simulink model "DSM_2"  (R2024b)
settings: Solver=VariableStepAuto  StartTime=0.0  StopTime=8e-3  RelTol=1e-3
undefined symbols (not defined in the file or in its folder): dspblkCoreblockFVToolHelper, gcbh
libraries: simulink x1
settings Model: Creator=peggy  LastModifiedBy=peggy

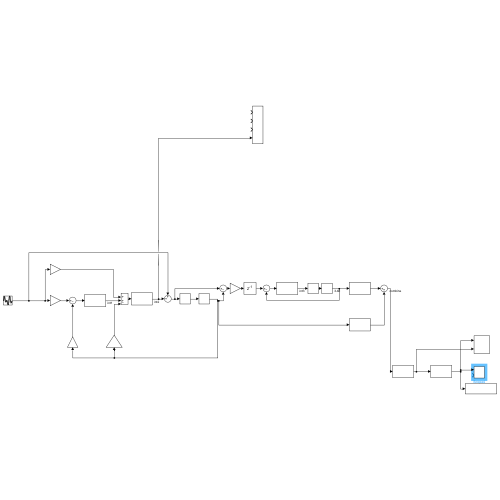
[thumbnail: Simulink's stored preview of the top-level diagram]
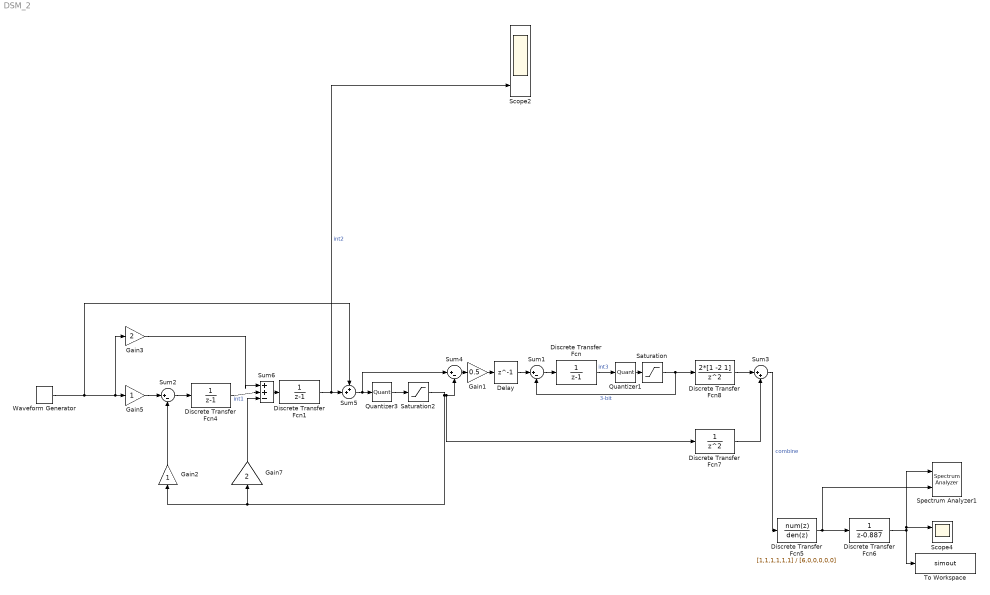
== system DSM_2 ==
  Delay : Delay  DelayLength=1  InitialCondition=0
  Discrete Transfer Fcn : DiscreteTransferFcn  LoadFcn=dspblkCoreblockFVToolHelper(gcbh,'load');  Denominator=[1 -1]
      settings: CopyFcn=dspblkCoreblockFVToolHelper(gcbh,'copy');  DeleteFcn=dspblkCoreblockFVToolHelper(gcbh,'close');  ModelCloseFcn=dspblkCoreblockFVToolHelper(gcbh,'close');  PreSaveFcn=dspblkCoreblockFVToolHelper(gcbh,'presave');  PostSaveFcn=dspblkCoreblockFVToolHelper(gcbh,'postsave');  CloseFcn=dspblkCoreblockFVToolHelper(gcbh,'close');
  Discrete Transfer Fcn1 : DiscreteTransferFcn  LoadFcn=dspblkCoreblockFVToolHelper(gcbh,'load');  Denominator=[1 -1]
      settings: CopyFcn=dspblkCoreblockFVToolHelper(gcbh,'copy');  DeleteFcn=dspblkCoreblockFVToolHelper(gcbh,'close');  ModelCloseFcn=dspblkCoreblockFVToolHelper(gcbh,'close');  PreSaveFcn=dspblkCoreblockFVToolHelper(gcbh,'presave');  PostSaveFcn=dspblkCoreblockFVToolHelper(gcbh,'postsave');  CloseFcn=dspblkCoreblockFVToolHelper(gcbh,'close');
  Discrete Transfer Fcn4 : DiscreteTransferFcn  LoadFcn=dspblkCoreblockFVToolHelper(gcbh,'load');  Denominator=[1 -1]
      settings: CopyFcn=dspblkCoreblockFVToolHelper(gcbh,'copy');  DeleteFcn=dspblkCoreblockFVToolHelper(gcbh,'close');  ModelCloseFcn=dspblkCoreblockFVToolHelper(gcbh,'close');  PreSaveFcn=dspblkCoreblockFVToolHelper(gcbh,'presave');  PostSaveFcn=dspblkCoreblockFVToolHelper(gcbh,'postsave');  CloseFcn=dspblkCoreblockFVToolHelper(gcbh,'close');
  Discrete Transfer Fcn5 : DiscreteTransferFcn  LoadFcn=dspblkCoreblockFVToolHelper(gcbh,'load');  Numerator=[1,1,1,1,1,1]  Denominator=[6,0,0,0,0,0]
      settings: CopyFcn=dspblkCoreblockFVToolHelper(gcbh,'copy');  DeleteFcn=dspblkCoreblockFVToolHelper(gcbh,'close');  ModelCloseFcn=dspblkCoreblockFVToolHelper(gcbh,'close');  PreSaveFcn=dspblkCoreblockFVToolHelper(gcbh,'presave');  PostSaveFcn=dspblkCoreblockFVToolHelper(gcbh,'postsave');  CloseFcn=dspblkCoreblockFVToolHelper(gcbh,'close');
  Discrete Transfer Fcn6 : DiscreteTransferFcn  LoadFcn=dspblkCoreblockFVToolHelper(gcbh,'load');  Denominator=[1 -0.887]
      settings: CopyFcn=dspblkCoreblockFVToolHelper(gcbh,'copy');  DeleteFcn=dspblkCoreblockFVToolHelper(gcbh,'close');  ModelCloseFcn=dspblkCoreblockFVToolHelper(gcbh,'close');  PreSaveFcn=dspblkCoreblockFVToolHelper(gcbh,'presave');  PostSaveFcn=dspblkCoreblockFVToolHelper(gcbh,'postsave');  CloseFcn=dspblkCoreblockFVToolHelper(gcbh,'close');
  Discrete Transfer Fcn7 : DiscreteTransferFcn  LoadFcn=dspblkCoreblockFVToolHelper(gcbh,'load');  Denominator=[1 0 0]
      settings: CopyFcn=dspblkCoreblockFVToolHelper(gcbh,'copy');  DeleteFcn=dspblkCoreblockFVToolHelper(gcbh,'close');  ModelCloseFcn=dspblkCoreblockFVToolHelper(gcbh,'close');  PreSaveFcn=dspblkCoreblockFVToolHelper(gcbh,'presave');  PostSaveFcn=dspblkCoreblockFVToolHelper(gcbh,'postsave');  CloseFcn=dspblkCoreblockFVToolHelper(gcbh,'close');
  Discrete Transfer Fcn8 : DiscreteTransferFcn  LoadFcn=dspblkCoreblockFVToolHelper(gcbh,'load');  Numerator=2*[1 -2 1]  Denominator=[1 0 0]
      settings: CopyFcn=dspblkCoreblockFVToolHelper(gcbh,'copy');  DeleteFcn=dspblkCoreblockFVToolHelper(gcbh,'close');  ModelCloseFcn=dspblkCoreblockFVToolHelper(gcbh,'close');  PreSaveFcn=dspblkCoreblockFVToolHelper(gcbh,'presave');  PostSaveFcn=dspblkCoreblockFVToolHelper(gcbh,'postsave');  CloseFcn=dspblkCoreblockFVToolHelper(gcbh,'close');
  Gain1 : Gain  Gain=0.5
  Gain2 : Gain
  Gain3 : Gain  Gain=2
  Gain5 : Gain
  Gain7 : Gain  Gain=2
  Quantizer1 : Quantizer  QuantizationInterval=1
  Quantizer3 : Quantizer  QuantizationInterval=1
  Saturation : Saturate  UpperLimit=1  LowerLimit=-1
  Saturation2 : Saturate  UpperLimit=1  LowerLimit=-1
  Scope2 : Scope  NumInputPorts=4
  Scope4 : Scope  NumInputPorts=2
  Spectrum Analyzer1 : SpectrumAnalyzer  NumInputPorts=2  WindowPosition=[-55.000000,159.000000,800.000000,500.000000,]  ScopeFrameLocation=window  WindowInvariantSamplesPerUpdate=on  Span=1000000  StartFrequency=-500000  StopFrequency=500000  YLimits=[-51.47127527,50.03311479]
  Sum1 : Sum  Inputs=|+-
  Sum2 : Sum  Inputs=|+-
  Sum3 : Sum  Inputs=|++
  Sum4 : Sum  Inputs=|+-
  Sum5 : Sum  Inputs=++|
  Sum6 : Sum  Inputs=|++-
  To Workspace : ToWorkspace  VariableName=simout  SaveFormat=Timeseries  SampleTime=-1
  Waveform Generator : simulink/Sources/Waveform Generator  OutMin=[]  OutMax=[]  OutDataTypeStr=double  SelectedSignal=1  Signals=sin(0.8,2e4,0)  BlockNames=MultiportSwitch_36150f93f18848f  SampleTime=1e-6
  wires:
  Sum2/1 -> Discrete Transfer Fcn4/1
  Sum3/1 -> Discrete Transfer Fcn5/1  "combine"
  Gain2/1 -> Sum2/2
  Discrete Transfer Fcn6/1 -> To Workspace/1, Spectrum Analyzer1/1, Scope4/1
  Waveform Generator/1 -> Sum5/1, Gain3/1, Gain5/1
  Gain5/1 -> Sum2/1
  Discrete Transfer Fcn5/1 -> Discrete Transfer Fcn6/1, Spectrum Analyzer1/2
  Saturation2/1 -> Discrete Transfer Fcn7/1, Sum4/2, Gain2/1, Gain7/1
  Discrete Transfer Fcn8/1 -> Sum3/1
  Sum6/1 -> Discrete Transfer Fcn1/1
  Quantizer3/1 -> Saturation2/1
  Quantizer1/1 -> Saturation/1
  Discrete Transfer Fcn/1 -> Quantizer1/1  "int3"
  Sum1/1 -> Discrete Transfer Fcn/1
  Saturation/1 -> Sum1/2, Discrete Transfer Fcn8/1  "3-bit"
  Delay/1 -> Sum1/1
  Discrete Transfer Fcn7/1 -> Sum3/2
  Sum4/1 -> Gain1/1
  Gain1/1 -> Delay/1
  Gain7/1 -> Sum6/3
  Discrete Transfer Fcn4/1 -> Sum6/2  "int1"
  Gain3/1 -> Sum6/1
  Sum5/1 -> Sum4/1, Quantizer3/1
  Discrete Transfer Fcn1/1 -> Scope2/4, Sum5/2  "int2"
